simulink model "model_example"  (R2023b)
settings: Solver=VariableStepAuto  StartTime=0.0  StopTime=10.0  FixedStep=0.0066666666666666671  MaxStep=0.1e-3
values from neighbouring files (symbols this model uses):
  fv = params(8)    [induction_motor.m]
  J = params(7)    [induction_motor.m]
  L_r = params(4)    [induction_motor.m]
  L_s = params(2)    [induction_motor.m]
  R_r = params(3)    [induction_motor.m]
  R_s = params(1)    [induction_motor.m]
libraries: eeTransforms x2, autolibim x1
settings Model: Creator=gosmann  LastModifiedBy=gosmann
settings SolverCC: MaxConsecutiveMinStep=100

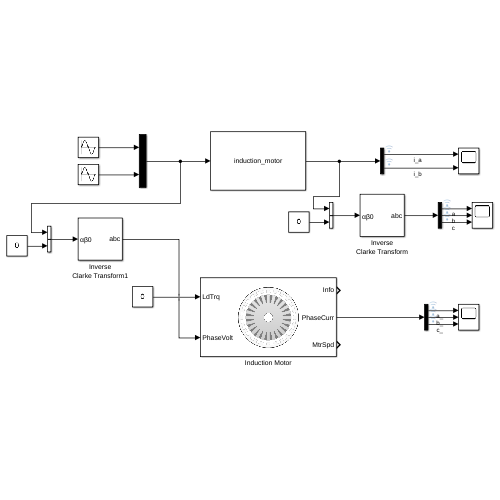
[thumbnail: Simulink's stored preview of the top-level diagram]
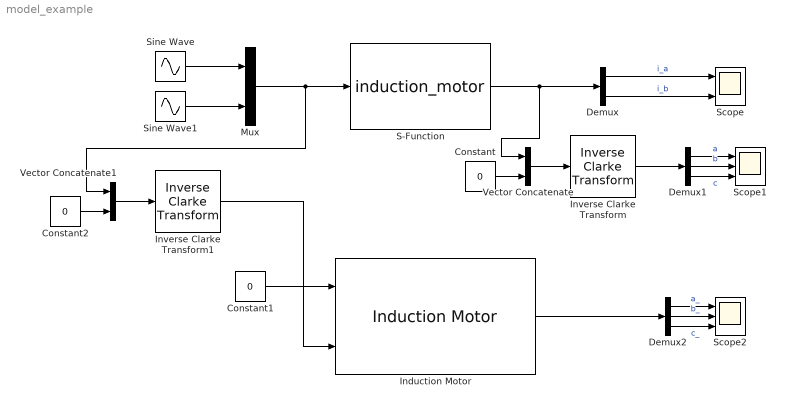
== system model_example ==
  Constant : Constant  Value=0
  Constant1 : Constant  Value=0
  Constant2 : Constant  Value=0
  Demux : Demux  Outputs=2
  Demux1 : Demux  Outputs=3
  Demux2 : Demux  Outputs=3
  Induction Motor : autolibim/Induction Motor  sim_type=Continuous  Ts=0.001  port_config=Torque  P=2  Zs=[R_s L_s]  Zr="[R_r  L_r]"  Lm=L_m  mechanical=[J fv 0]  theta_init=0  omega_init=0  RefBlkName='autolibim/Induction Motor'  aMode=1
      settings: LibrarySourceBlock=autolibemachines/Induction Motor
  Inverse Clarke Transform : eeTransforms/Inverse Clarke Transform  PowerInvariant=off
      settings: LibrarySourceBlock=|
      | ee_sl_lib/Mathematical
      | Transforms/Inverse
      | Clarke Transform
  Inverse Clarke Transform1 : eeTransforms/Inverse Clarke Transform  PowerInvariant=on
      settings: LibrarySourceBlock=|
      | ee_sl_lib/Mathematical
      | Transforms/Inverse
      | Clarke Transform
  Mux : Mux  Inputs=2
  S-Function : S-Function  FunctionName=induction_motor  Parameters=params  SFunctionDeploymentMode=off  EnableBusSupport=off
  Scope : Scope  NumInputPorts=2
  Scope1 : Scope  NumInputPorts=3
  Scope2 : Scope  NumInputPorts=3
  Sine Wave : Sin  Amplitude=100  Frequency=2*pi*50  SampleTime=0
  Sine Wave1 : Sin  Amplitude=100  Frequency=2*pi*50  Phase=0+(pi/180)*90  SampleTime=0
  Vector Concatenate : Concatenate
  Vector Concatenate1 : Concatenate
  wires:
  Sine Wave/1 -> Mux/1
  Sine Wave1/1 -> Mux/2
  S-Function/1 -> Vector Concatenate/1, Demux/1
  Demux/2 -> Scope/2  "i_b"
  Demux/1 -> Scope/1  "i_a"
  Inverse Clarke Transform/1 -> Demux1/1
  Demux1/1 -> Scope1/1  "a"
  Demux1/2 -> Scope1/2  "b"
  Demux1/3 -> Scope1/3  "c"
  Vector Concatenate/1 -> Inverse Clarke Transform/1
  Constant/1 -> Vector Concatenate/2
  Demux2/2 -> Scope2/2  "b_"
  Demux2/3 -> Scope2/3  "c_"
  Induction Motor/2 -> Demux2/1
  Demux2/1 -> Scope2/1  "a_"
  Constant1/1 -> Induction Motor/1
  Mux/1 -> Vector Concatenate1/1, S-Function/1
  Vector Concatenate1/1 -> Inverse Clarke Transform1/1
  Constant2/1 -> Vector Concatenate1/2
  Inverse Clarke Transform1/1 -> Induction Motor/2
